simulink model "PlannedIsland_Harness"  (R2025b)
settings: Solver=FixedStepAuto  StartTime=0.0  StopTime=20  RelTol=1e-3
PostLoadFcn:
  | PlannedIslandParam;
values from neighbouring files (symbols this model uses):
  Ts = 5E-5    (= 5e-05)    [BESSGFLParam.m]    (also in BESSGFMParam.m; WindFarmParam.m)
undefined symbols (not defined in the file or in its folder): plannedIsland
libraries: slpidlib x2, eeGeneralControl x1
settings Model: Creator=skota  LastModifiedBy=skota

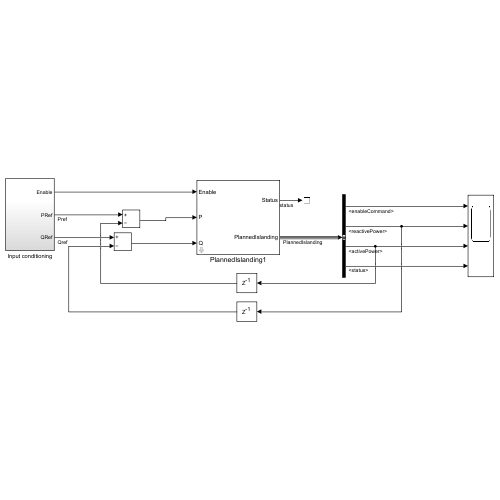
[thumbnail: Simulink's stored preview of the top-level diagram]
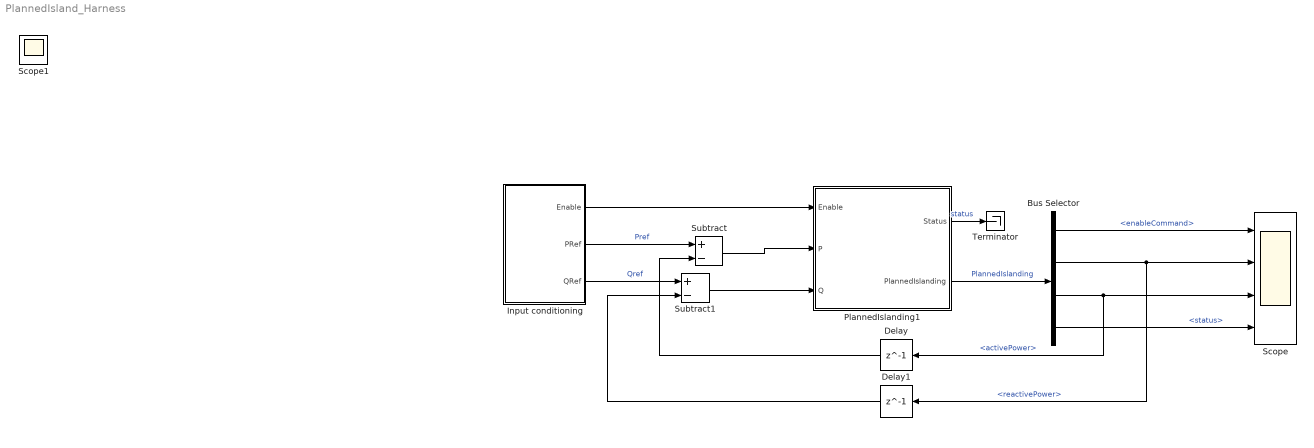
== system PlannedIsland_Harness ==
  Bus Selector : BusSelector  OutputSignals=enableCommand,reactivePower,activePower,status
  Delay : Delay  DelayLength=1
  Delay1 : Delay  DelayLength=1
  Input conditioning : Subsystem
  PlannedIslanding1 : Subsystem  mask(PlannedIslanding){KpPPlannedIsland=plannedIsland.kPActive, KiPPlannedIsland=plannedIsland.kIActive, ZeroActivePowerThreshold=plannedIsland.pThreshold, KpQPlannedIsland=plannedIsland.kPReactive, KiQPlannedIsland=plannedIsland.kiReactive, ZeroReactivePowerThreshold=plannedIsland.qThreshold}
      mask prompts: KpPPlannedIsland "Proportional Gain"; KiPPlannedIsland "Integral Gain"; ZeroActivePowerThreshold "Threshold"; KpQPlannedIsland "Proportional Gain"; KiQPlannedIsland "Integral Gain"; ZeroReactivePowerThreshold "Threshold"
      mask help: This block enables the microgrid to island from the grid in a planned manner by reducing the active and reactive power from the grid
      settings: CopyFcn=set_param(gcbh,'LinkStatus','none');
      mask Help: web('PlannedIslanding.html')
      mask DialogControl Container4 Prompt: Active Power
      mask DialogControl Container5 Prompt: Reactive Power
  Scope : Scope  NumInputPorts=4
      settings: ActiveDisplayYMinimum=-0.12499999999999997  ActiveDisplayYMaximum=1.125
  Subtract : Sum  Inputs=+-
  Subtract1 : Sum  Inputs=+-
  Terminator : Terminator
  Scope1 : Scope
      settings: DataLoggingVariableName=ScopeData3
  wires:
  Input conditioning/2(PRef) -> Subtract/1  "Pref"
  Bus Selector/1 -> Scope/1  "<enableCommand>"
  Bus Selector/2 -> Delay1/1, Scope/2  "<reactivePower>"
  Input conditioning/3(QRef) -> Subtract1/1  "Qref"
  PlannedIslanding1/1(Status) -> Terminator/1  "status"
  Delay1/1 -> Subtract1/2
  Subtract/1 -> PlannedIslanding1/2(P)
  Input conditioning/1(Enable) -> PlannedIslanding1/1(Enable)
  PlannedIslanding1/2(PlannedIslanding) -> Bus Selector/1  "PlannedIslanding"
  Bus Selector/3 -> Delay/1, Scope/3  "<activePower>"
  Bus Selector/4 -> Scope/4  "<status>"
  Delay/1 -> Subtract/2
  Subtract1/1 -> PlannedIslanding1/3(Q)

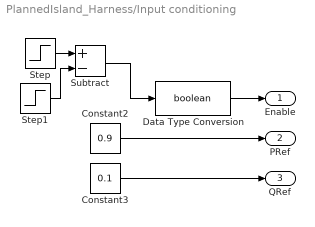
== system PlannedIsland_Harness/Input conditioning ==
  Constant2 : Constant  Value=0.9
  Constant3 : Constant  Value=0.1
  Data Type Conversion : DataTypeConversion  OutDataTypeStr=boolean  SaturateOnIntegerOverflow=off  RndMeth=Floor
  Step : Step  Time=3  SampleTime=0
  Step1 : Step  Time=12  SampleTime=0
  Subtract : Sum  Inputs=+-
  Enable : Outport
  PRef : Outport  Port=2
  QRef : Outport  Port=3
  wires:
  Constant2/1 -> PRef/1
  Constant3/1 -> QRef/1
  Data Type Conversion/1 -> Enable/1
  Subtract/1 -> Data Type Conversion/1
  Step/1 -> Subtract/1
  Step1/1 -> Subtract/2

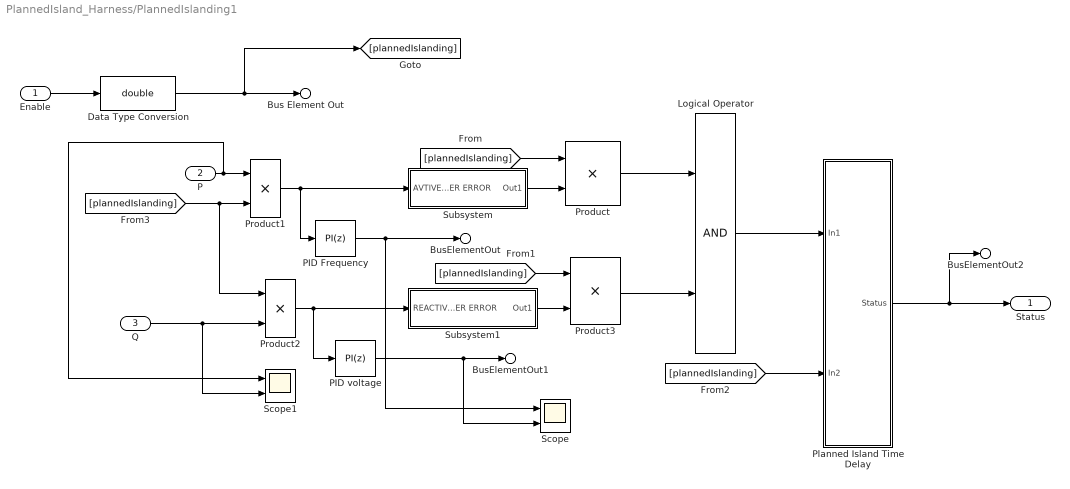
== system PlannedIsland_Harness/PlannedIslanding1 ==
  Enable : Inport
  P : Inport  Port=2
  Q : Inport  Port=3
  Data Type Conversion : DataTypeConversion  OutDataTypeStr=double  SaturateOnIntegerOverflow=off  RndMeth=Floor
  Logical Operator : Logic  AllPortsSameDT=off  OutDataTypeStr=boolean
  PID Frequency : slpidlib/PID Controller  Controller=PI  Form=Parallel  TimeDomain=Discrete-time  UseExternalTs=off  SampleTime=Ts  IntegratorMethod=Forward Euler  FilterMethod=Forward Euler  ControllerParametersSource=internal  P=KpPPlannedIsland  I=KiPPlannedIsland  UseKiTs=off  D=0  UseExternalDerivativeSource=off  N=100  UseFilter=on  TunerSelectOption=Frequency Response Based  InitialConditionSource=internal  InitialConditionForIntegrator=0  InitialConditionForFilter=0  DifferentiatorICPrevScaledInput=0  ExternalReset=none  TrackingMode=off  Kt=1  LimitOutput=off  SatLimitsSource=internal  UpperSaturationLimit=0.05  LowerSaturationLimit=-0.05  LinearizeAsGain=on  AntiWindupMode=clamping  Kb=1  LimitIntegrator=off  UpperIntegratorSaturationLimit=inf  LowerIntegratorSaturationLimit=-inf  POutMin=[]  POutMax=[]  IOutMin=[]  IOutMax=[]  DOutMin=[]  DOutMax=[]  NOutMin=[]  NOutMax=[]  SumOutMin=[]  SumOutMax=[]  SaturationOutMin=[]  SaturationOutMax=[]  PParamMin=[]  PParamMax=[]  IParamMin=[]  IParamMax=[]  DParamMin=[]  DParamMax=[]  NParamMin=[]  NParamMax=[]  KbParamMin=[]  KbParamMax=[]  KtParamMin=[]  KtParamMax=[]  KbOutMin=[]  KbOutMax=[]  KtOutMin=[]  KtOutMax=[]  IntegratorOutMin=[]  IntegratorOutMax=[]  FilterOutMin=[]  FilterOutMax=[]  SumI1OutMin=[]  SumI1OutMax=[]  SumI2OutMin=[]  SumI2OutMax=[]  SumI3OutMin=[]  SumI3OutMax=[]  SumI4OutMin=[]  SumI4OutMax=[]  SumDOutMin=[]  SumDOutMax=[]  DifferentiatorOutMin=[]  DifferentiatorOutMax=[]  FilterDiffOutCoefMin=[]  FilterDiffOutCoefMax=[]  ReciprocalOutMin=[]  ReciprocalOutMax=[]  SumDenOutMin=[]  SumDenOutMax=[]  SumNumOutMin=[]  SumNumOutMax=[]  DivideOutMin=[]  DivideOutMax=[]  UdiffTsProdOutMin=[]  UdiffTsProdOutMax=[]  NTsProdOutMin=[]  NTsProdOutMax=[]  UintegralTsProdOutMin=[]  UintegralTsProdOutMax=[]  UngainTsProdOutMin=[]  UngainTsProdOutMax=[]  ClampingZeroOutDataTypeStr=Inherit: Inherit via back propagation  ClampingZeroOutMin=[]  ClampingZeroOutMax=[]  FilterDenConstantOutDataTypeStr=Inherit: Inherit via back propagation  FilterDenConstantOutMin=[]  FilterDenConstantOutMax=[]  PCopyOutDataTypeStr=Inherit: Inherit via back propagation  PCopyOutMin=[]  PCopyOutMax=[]  NCopyOutDataTypeStr=Inherit: Inherit via back propagation  NCopyOutMin=[]  NCopyOutMax=[]  IntegratorContinuousStateAttributes=''  IntegratorStateMustResolveToSignalObject=off  IntegratorRTWStateStorageClass=Auto  FilterContinuousStateAttributes=''  FilterStateMustResolveToSignalObject=off  FilterRTWStateStorageClass=Auto  ParallelPVariant=InternalParameters  IdealPVariant=Disabled  IVariant=InternalParameters  DVariant=Disabled  IntegratorVariant=Discrete  SatVariant=Disabled  AWVariant=Passthrough  PCopyVariant=Disabled  TRVariant=Disabled  FdbkBlocksVariant=Forward  IdealPFdbkVariant=Disabled  SatFdbkVariant=Disabled  DerivativeFilterVariant=Disabled  NVariant=Disabled  NCopyVariant=Disabled_SignalSpec  FilterICVariant=Disabled  IntegratorICVariant=InternalICs  ExternalResetVariant=Disabled  TRSumVariant=Passthrough  SumFdbkVariant=Disabled  SumVariant=Sum_PI  TsampFilterVariant=InternalTs  TsampNgainVariant=Passthrough  TsampIntegralVariant=Disabled_SignalSpec  ExternalSaturationOutDataTypeStr=Inherit: Same as second input  DerivativeSourceVariant=Disabled  PreIntVariant=InternalPreInt
  PID voltage : slpidlib/PID Controller  Controller=PI  Form=Parallel  TimeDomain=Discrete-time  UseExternalTs=off  SampleTime=Ts  IntegratorMethod=Forward Euler  FilterMethod=Forward Euler  ControllerParametersSource=internal  P=KpQPlannedIsland  I=KiQPlannedIsland  UseKiTs=off  D=0  UseExternalDerivativeSource=off  N=100  UseFilter=on  TunerSelectOption=Frequency Response Based  InitialConditionSource=internal  InitialConditionForIntegrator=0  InitialConditionForFilter=0  DifferentiatorICPrevScaledInput=0  ExternalReset=none  TrackingMode=off  Kt=1  LimitOutput=off  SatLimitsSource=internal  UpperSaturationLimit=0.05  LowerSaturationLimit=-0.05  LinearizeAsGain=on  AntiWindupMode=clamping  Kb=1  LimitIntegrator=off  UpperIntegratorSaturationLimit=inf  LowerIntegratorSaturationLimit=-inf  POutMin=[]  POutMax=[]  IOutMin=[]  IOutMax=[]  DOutMin=[]  DOutMax=[]  NOutMin=[]  NOutMax=[]  SumOutMin=[]  SumOutMax=[]  SaturationOutMin=[]  SaturationOutMax=[]  PParamMin=[]  PParamMax=[]  IParamMin=[]  IParamMax=[]  DParamMin=[]  DParamMax=[]  NParamMin=[]  NParamMax=[]  KbParamMin=[]  KbParamMax=[]  KtParamMin=[]  KtParamMax=[]  KbOutMin=[]  KbOutMax=[]  KtOutMin=[]  KtOutMax=[]  IntegratorOutMin=[]  IntegratorOutMax=[]  FilterOutMin=[]  FilterOutMax=[]  SumI1OutMin=[]  SumI1OutMax=[]  SumI2OutMin=[]  SumI2OutMax=[]  SumI3OutMin=[]  SumI3OutMax=[]  SumI4OutMin=[]  SumI4OutMax=[]  SumDOutMin=[]  SumDOutMax=[]  DifferentiatorOutMin=[]  DifferentiatorOutMax=[]  FilterDiffOutCoefMin=[]  FilterDiffOutCoefMax=[]  ReciprocalOutMin=[]  ReciprocalOutMax=[]  SumDenOutMin=[]  SumDenOutMax=[]  SumNumOutMin=[]  SumNumOutMax=[]  DivideOutMin=[]  DivideOutMax=[]  UdiffTsProdOutMin=[]  UdiffTsProdOutMax=[]  NTsProdOutMin=[]  NTsProdOutMax=[]  UintegralTsProdOutMin=[]  UintegralTsProdOutMax=[]  UngainTsProdOutMin=[]  UngainTsProdOutMax=[]  ClampingZeroOutDataTypeStr=Inherit: Inherit via back propagation  ClampingZeroOutMin=[]  ClampingZeroOutMax=[]  FilterDenConstantOutDataTypeStr=Inherit: Inherit via back propagation  FilterDenConstantOutMin=[]  FilterDenConstantOutMax=[]  PCopyOutDataTypeStr=Inherit: Inherit via back propagation  PCopyOutMin=[]  PCopyOutMax=[]  NCopyOutDataTypeStr=Inherit: Inherit via back propagation  NCopyOutMin=[]  NCopyOutMax=[]  IntegratorContinuousStateAttributes=''  IntegratorStateMustResolveToSignalObject=off  IntegratorRTWStateStorageClass=Auto  FilterContinuousStateAttributes=''  FilterStateMustResolveToSignalObject=off  FilterRTWStateStorageClass=Auto  ParallelPVariant=InternalParameters  IdealPVariant=Disabled  IVariant=InternalParameters  DVariant=Disabled  IntegratorVariant=Discrete  SatVariant=Disabled  AWVariant=Passthrough  PCopyVariant=Disabled  TRVariant=Disabled  FdbkBlocksVariant=Forward  IdealPFdbkVariant=Disabled  SatFdbkVariant=Disabled  DerivativeFilterVariant=Disabled  NVariant=Disabled  NCopyVariant=Disabled_SignalSpec  FilterICVariant=Disabled  IntegratorICVariant=InternalICs  ExternalResetVariant=Disabled  TRSumVariant=Passthrough  SumFdbkVariant=Disabled  SumVariant=Sum_PI  TsampFilterVariant=InternalTs  TsampNgainVariant=Passthrough  TsampIntegralVariant=Disabled_SignalSpec  ExternalSaturationOutDataTypeStr=Inherit: Same as second input  DerivativeSourceVariant=Disabled  PreIntVariant=InternalPreInt
  Planned Island Time Delay : Subsystem
  Product{,1..3} (4 alike) : Product
  Scope : Scope  NumInputPorts=2
      settings: ActiveDisplayYMinimum=-1  ActiveDisplayYMaximum=1  DataLoggingVariableName=ScopeData35
  Scope1 : Scope  NumInputPorts=2
      settings: ActiveDisplayYMinimum=-1.6827967094302978  ActiveDisplayYMaximum=1.1685546180291482  DataLoggingVariableName=ScopeData36
  Subsystem : Subsystem
  Subsystem1 : Subsystem
  Status : Outport
  Bus Element Out : Outport  Port=2  PortName=PlannedIslanding  Element=enableCommand
  BusElementOut : Outport  Port=2  PortName=PlannedIslanding  Element=activePower
  BusElementOut1 : Outport  Port=2  PortName=PlannedIslanding  Element=reactivePower
  BusElementOut2 : Outport  Port=2  PortName=PlannedIslanding  Element=status
  wires:
  ? -> ?
  Data Type Conversion/1 -> [plannedIslanding], Bus Element Out/1
  Product2/1 -> Subsystem1/1(REACTIVEPOWER ERROR), PID voltage/1
  Enable/1 -> Data Type Conversion/1
  Logical Operator/1 -> Planned Island Time Delay/1(In1)
  P/1 -> Product1/1, Scope1/1
  Subsystem/1(Out1) -> Product/2
  [plannedIslanding] -> Product2/1, Product1/2
  Subsystem1/1(Out1) -> Product3/2
  Q/1 -> Product2/2, Scope1/2
  Product/1 -> Logical Operator/1
  Planned Island Time Delay/1(Status) -> Status/1, BusElementOut2/1
  PID Frequency/1 -> Scope/1, BusElementOut/1
  [plannedIslanding] -> Product/1
  [plannedIslanding] -> Planned Island Time Delay/2(In2)
  [plannedIslanding] -> Product3/1
  PID voltage/1 -> BusElementOut1/1, Scope/2
  Product3/1 -> Logical Operator/2
  Product1/1 -> PID Frequency/1, Subsystem/1(AVTIVE POWER ERROR)

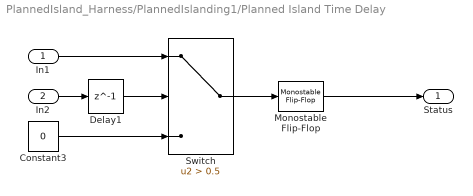
== system PlannedIsland_Harness/PlannedIslanding1/Planned Island Time Delay ==
  In1 : Inport
  In2 : Inport  Port=2
  Constant3 : Constant  Value=0
  Delay1 : Delay  DelayLength=1  SampleTime=Ts
  Monostable Flip-Flop : eeGeneralControl/Monostable Flip-Flop  VariantControl=Variant1  LabelModeActiveChoice=Discrete  ChangeType=Rising edge  x0=0  Td=100  Ts=Ts
  Switch : Switch  Criteria=u2 > Threshold  Threshold=0.5  SaturateOnIntegerOverflow=off  InputSameDT=off
  Status : Outport
  wires:
  In2/1 -> Delay1/1
  In1/1 -> Switch/1
  Monostable Flip-Flop/1 -> Status/1
  Delay1/1 -> Switch/2
  Constant3/1 -> Switch/3
  Switch/1 -> Monostable Flip-Flop/1

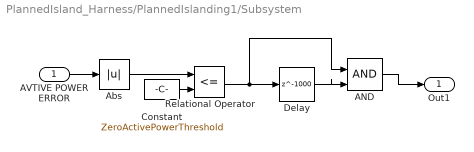
== system PlannedIsland_Harness/PlannedIslanding1/Subsystem ==
  AVTIVE POWER ERROR : Inport
  AND : Logic  IconShape=distinctive  AllPortsSameDT=off  OutDataTypeStr=boolean
  Abs : Abs  SaturateOnIntegerOverflow=off
  Constant : Constant  Value=ZeroActivePowerThreshold  SampleTime=-1
  Delay : Delay  DelayLength=1000  SampleTime=Ts
  Relational Operator : RelationalOperator  Operator=<=  OutDataTypeStr=boolean  RndMeth=Simplest  InputSameDT=off
  Out1 : Outport
  wires:
  Delay/1 -> AND/2
  Constant/1 -> Relational Operator/2
  Relational Operator/1 -> AND/1, Delay/1
  AND/1 -> Out1/1
  AVTIVE POWER ERROR/1 -> Abs/1
  Abs/1 -> Relational Operator/1

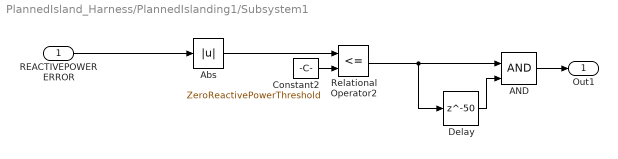
== system PlannedIsland_Harness/PlannedIslanding1/Subsystem1 ==
  REACTIVEPOWER ERROR : Inport
  AND : Logic  IconShape=distinctive  AllPortsSameDT=off  OutDataTypeStr=boolean
  Abs : Abs  SaturateOnIntegerOverflow=off
  Constant2 : Constant  Value=ZeroReactivePowerThreshold
  Delay : Delay  DelayLength=50  SampleTime=Ts
  Relational Operator2 : RelationalOperator  Operator=<=  OutDataTypeStr=boolean  RndMeth=Simplest  InputSameDT=off
  Out1 : Outport
  wires:
  Delay/1 -> AND/2
  REACTIVEPOWER ERROR/1 -> Abs/1
  Relational Operator2/1 -> Delay/1, AND/1
  Constant2/1 -> Relational Operator2/2
  AND/1 -> Out1/1
  Abs/1 -> Relational Operator2/1
